simulink model "HANcoder_E407_GTSync_v3_clean"  (R2018b)
settings: Solver=FixedStepDiscrete  StartTime=0.0  StopTime=1  FixedStep=0.01  RelTol=1e-3
PreLoadFcn:
  | librarySetup
  | eval([bdroot,'_startup']) %Calling [modelName]_startup.m
values from neighbouring files (symbols this model uses):
  basic_cycle_duration = 60000    [HANcoder_E407_GTSync_v3_clean_startup.m]    (also in HANcoder_E407_GTSync_v3_startup.m = 50000)
  comm_delay_estimation = 3    [HANcoder_E407_GTSync_v3_clean_startup.m]
  frequency_IRQ = 100    [HANcoder_E407_GTSync_startup.m]    (also in HANcoder_E407_GTSync_v3_clean_startup.m = 99; HANcoder_E407_GTSync_v3_startup.m = 99)
  HANtuneOverride = Simulink.Parameter    [HANcoder_E407_GTSync_startup.m]    (also in HANcoder_E407_GTSync_v3_clean_startup.m; HANcoder_E407_GTSync_v3_startup.m)
  LED_ticks_toggle = 10000    [HANcoder_E407_GTSync_startup.m]    (also in HANcoder_E407_GTSync_v3_clean_startup.m; HANcoder_E407_GTSync_v3_startup.m)
  Master_Role = 1    [HANcoder_E407_GTSync_v3_clean_startup.m]    (also in HANcoder_E407_GTSync_v3_startup.m)
  matrix_rows = 2    [HANcoder_E407_GTSync_v3_clean_startup.m]    (also in HANcoder_E407_GTSync_v3_startup.m)
  Slave_Role = 2    [HANcoder_E407_GTSync_v3_clean_startup.m]    (also in HANcoder_E407_GTSync_v3_startup.m)
  Sync_ID = 1    [HANcoder_E407_GTSync_v3_clean_startup.m]    (also in HANcoder_E407_GTSync_v3_startup.m)
  time_difference_threshold = 500    [HANcoder_E407_GTSync_v3_clean_startup.m]    (also in HANcoder_E407_GTSync_v3_startup.m = 100)
  TM0 = 100    [HANcoder_E407_GTSync_v3_clean_startup.m]    (also in HANcoder_E407_GTSync_v3_startup.m = 0)
  TM1 = 20000    [HANcoder_E407_GTSync_v3_clean_startup.m]    (also in HANcoder_E407_GTSync_v3_startup.m = 25000)
  TM2 = 30000    [HANcoder_E407_GTSync_v3_clean_startup.m]    (also in HANcoder_E407_GTSync_v3_startup.m = 37500)
  TM3 = 40000    [HANcoder_E407_GTSync_v3_clean_startup.m]    (also in HANcoder_E407_GTSync_v3_startup.m)
  TM4 = 50000    [HANcoder_E407_GTSync_v3_clean_startup.m]
  Vote1_ID = 12    [HANcoder_E407_GTSync_v3_clean_startup.m]    (also in HANcoder_E407_GTSync_v3_startup.m)
  Vote2_ID = 22    [HANcoder_E407_GTSync_v3_clean_startup.m]    (also in HANcoder_E407_GTSync_v3_startup.m)
  Vote3_ID = 32    [HANcoder_E407_GTSync_v3_clean_startup.m]    (also in HANcoder_E407_GTSync_v3_startup.m)
  wrap_up_threshold = basic_cycle_duration - time_difference_threshold*10    (= 55000)    [HANcoder_E407_GTSync_v3_clean_startup.m]
libraries: HANcoder_STM32_Target x20, simulink x3, simulink_extras x1
(part 3 of 4)

== system HANcoder_E407_GTSync_v3_clean/HANcoder STM32 Target - E407-STM32 algorithm/Global Ticks Increment/CAN Management/CAN Recieve/CAN Receive System/Subsystem3 ==
  Enable : EnablePort
  Bus Creator : BusCreator  Inputs=9
  CAN receive : Subsystem  Tag=HANcoder_TARGET_STM32_E407  AncestorBlock=HANcoder_STM32_Target/STM32-E407/CAN/CAN/CAN receive  mask(CAN receive){canBus=CAN 2, outputNumber=8, dataType=uint8, byteOrder=off, tsamp=-1}
      mask prompts: canBus "CAN channel"; outputNumber "Output ports"; dataType "Output datatype"; byteOrder "Byte order: Checked = MSB first, unchecked = LSB first."; tsamp "Sample time"
      mask help:
      | Function
      | ==========
      | Receive the newest message from the specified CAN channel.
      |
      | Parameters
      | ==========
      | CAN channel:             The CAN channel to send the message on.
      | Output ports:             The amount of output ports
      | Output datatype:       The datatype of the output ports
      | Byte order:                 Select MSB or LSB first
      | Sample time:              -1 or divisible by base sample time [seconds]
      |
      | Input
      | ==========
      | Port 1:                       CAN ID(uint32) in hexadecimal ie: hex2dec('0a')
      |
      | Output
      | ==========
      | Port 1:                       Checks for new message(int8)
      | Port 2..9                     Message data
      mask init:
      | sfcn_can_receive_mcb(canBus, outputNumber, dataType, byteOrder)
      settings: MoveFcn=drawLogos
      mask Help: web('sfcn_can_receive.html');
      mask TypeOptions canBus: CAN 1 | CAN 2
      mask TypeOptions dataType: int8 | uint8 | int16 | uint16 | int32 | uint32 | boolean
      mask Display:
      | fprintf('Receive on\nCAN %x', canBus);
      | port_label('output', 1, 'new');
      | port_label('input', 1, 'ID');patch([85 91 91],[8 14 2],[1 0 0]);patch([93 93 99],[14 2 8],[0 0 0.35]);
  Constant4 : Constant  Value=Vote3_ID  OutDataTypeStr=uint32
  Output : Outport
  wires:
  Constant4/1 -> CAN receive/1(In1)
  Bus Creator/1 -> Output/1
  CAN receive/1(Out1) -> Bus Creator/1
  CAN receive/9(Out9) -> Bus Creator/9
  CAN receive/8(Out8) -> Bus Creator/8
  CAN receive/7(Out7) -> Bus Creator/7
  CAN receive/6(Out6) -> Bus Creator/6
  CAN receive/5(Out5) -> Bus Creator/5
  CAN receive/4(Out4) -> Bus Creator/4
  CAN receive/3(Out3) -> Bus Creator/3
  CAN receive/2(Out2) -> Bus Creator/2

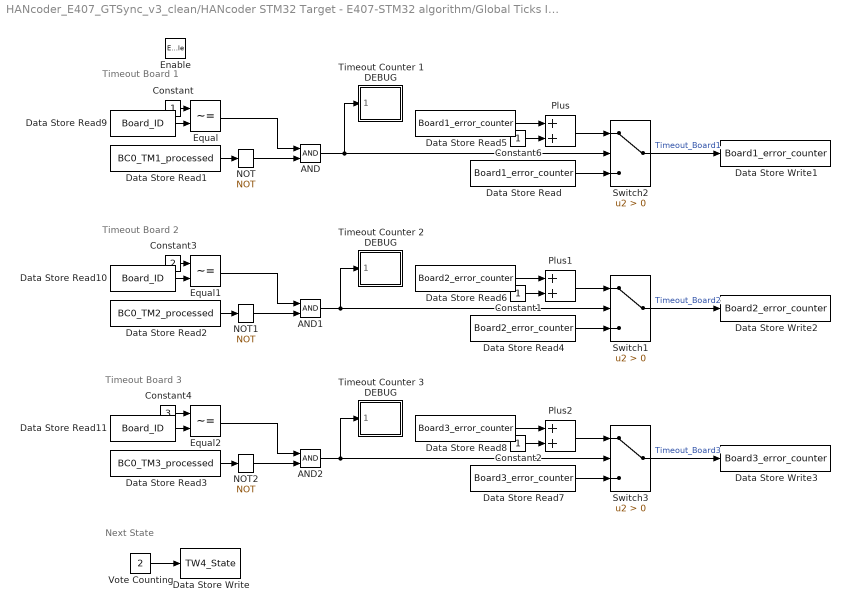
== system HANcoder_E407_GTSync_v3_clean/HANcoder STM32 Target - E407-STM32 algorithm/Global Ticks Increment/CAN Management/Matrix Cycle Manager/BC0 TW4/Subsystem ==
  note: Timeout Board 3
  note: Timeout Board 2
  note: Timeout Board 1
  note: Next State
  Enable : EnablePort
  AND : Logic  IconShape=distinctive  AllPortsSameDT=off  OutDataTypeStr=boolean
  AND1 : Logic  IconShape=distinctive  AllPortsSameDT=off  OutDataTypeStr=boolean
  AND2 : Logic  IconShape=distinctive  AllPortsSameDT=off  OutDataTypeStr=boolean
  Constant{,1..2,6} (4 alike) : Constant
  Constant3 : Constant  Value=2
  Constant4 : Constant  Value=3
  Data Store Read : DataStoreRead  DataStoreName=Board1_error_counter
  Data Store Read1 : DataStoreRead  DataStoreName=BC0_TM1_processed
  Data Store Read10 : DataStoreRead  DataStoreName=Board_ID
  Data Store Read11 : DataStoreRead  DataStoreName=Board_ID
  Data Store Read2 : DataStoreRead  DataStoreName=BC0_TM2_processed
  Data Store Read3 : DataStoreRead  DataStoreName=BC0_TM3_processed
  Data Store Read4 : DataStoreRead  DataStoreName=Board2_error_counter
  Data Store Read5 : DataStoreRead  DataStoreName=Board1_error_counter
  Data Store Read6 : DataStoreRead  DataStoreName=Board2_error_counter
  Data Store Read7 : DataStoreRead  DataStoreName=Board3_error_counter
  Data Store Read8 : DataStoreRead  DataStoreName=Board3_error_counter
  Data Store Read9 : DataStoreRead  DataStoreName=Board_ID
  Data Store Write : DataStoreWrite  DataStoreName=TW4_State
  Data Store Write1 : DataStoreWrite  DataStoreName=Board1_error_counter
  Data Store Write2 : DataStoreWrite  DataStoreName=Board2_error_counter
  Data Store Write3 : DataStoreWrite  DataStoreName=Board3_error_counter
  Equal : RelationalOperator  Operator=~=  OutDataTypeStr=boolean  RndMeth=Simplest
  Equal1 : RelationalOperator  Operator=~=  OutDataTypeStr=boolean  RndMeth=Simplest
  Equal2 : RelationalOperator  Operator=~=  OutDataTypeStr=boolean  RndMeth=Simplest
  NOT : Logic  Operator=NOT  IconShape=distinctive  AllPortsSameDT=off  OutDataTypeStr=boolean
  NOT1 : Logic  Operator=NOT  IconShape=distinctive  AllPortsSameDT=off  OutDataTypeStr=boolean
  NOT2 : Logic  Operator=NOT  IconShape=distinctive  AllPortsSameDT=off  OutDataTypeStr=boolean
  Plus : Sum
  Plus1 : Sum
  Plus2 : Sum
  Switch1 : Switch  Criteria=u2 > Threshold
  Switch2 : Switch  Criteria=u2 > Threshold
  Switch3 : Switch  Criteria=u2 > Threshold
  Timeout Counter 1 DEBUG : Subsystem
  Timeout Counter 2 DEBUG : Subsystem
  Timeout Counter 3 DEBUG : Subsystem
  Vote Counting : Constant  Value=2
  wires:
  Vote Counting/1 -> Data Store Write/1
  Constant6/1 -> Plus/2
  Plus/1 -> Switch2/1
  Data Store Read5/1 -> Plus/1
  Switch2/1 -> Data Store Write1/1  "Timeout_Board1"
  Data Store Read/1 -> Switch2/3
  Data Store Read1/1 -> NOT/1
  Data Store Read2/1 -> NOT1/1
  Data Store Read4/1 -> Switch1/3
  Switch1/1 -> Data Store Write2/1  "Timeout_Board2"
  Data Store Read6/1 -> Plus1/1
  Plus1/1 -> Switch1/1
  Constant1/1 -> Plus1/2
  Constant2/1 -> Plus2/2
  Plus2/1 -> Switch3/1
  Switch3/1 -> Data Store Write3/1  "Timeout_Board3"
  Data Store Read7/1 -> Switch3/3
  Data Store Read3/1 -> NOT2/1
  Data Store Read8/1 -> Plus2/1
  NOT/1 -> AND/2
  Data Store Read9/1 -> Equal/2
  Constant/1 -> Equal/1
  Equal/1 -> AND/1
  AND/1 -> Timeout Counter 1 DEBUG/1(Timeout), Switch2/2
  Equal1/1 -> AND1/1
  Equal2/1 -> AND2/1
  NOT2/1 -> AND2/2
  AND2/1 -> Timeout Counter 3 DEBUG/1(Timeout), Switch3/2
  Data Store Read11/1 -> Equal2/2
  Constant4/1 -> Equal2/1
  Data Store Read10/1 -> Equal1/2
  Constant3/1 -> Equal1/1
  AND1/1 -> Timeout Counter 2 DEBUG/1(Timeout), Switch1/2
  NOT1/1 -> AND1/2

== system HANcoder_E407_GTSync_v3_clean/HANcoder STM32 Target - E407-STM32 algorithm/Global Ticks Increment/CAN Management/Matrix Cycle Manager/BC0 TW4/Subsystem2 ==
  note: Next State
  note: Post voting process
  Enable : EnablePort  PropagateVarSize=During execution
  Constant10 : Constant  Value=Slave_Role
  Constant9 : Constant  Value=Master_Role
  Data Store Read : DataStoreRead  DataStoreName=Master_ID
  Data Store Read27 : DataStoreRead  DataStoreName=Board_ID
  Data Store Write : DataStoreWrite  DataStoreName=TW4_State
  Data Store Write1 : DataStoreWrite  DataStoreName=New_Master
  Data Store Write13 : DataStoreWrite  DataStoreName=Master_ID
  Data Store Write15 : DataStoreWrite  DataStoreName=Role_ID
  Equal : RelationalOperator  Operator=~=  OutDataTypeStr=boolean  RndMeth=Simplest
  Equal6 : RelationalOperator  Operator===  OutDataTypeStr=boolean  RndMeth=Simplest
  RESET Board - Return to initialization : Subsystem  TreatAsAtomicUnit=on
  Reset Variables : Constant  Value=3
  Switch16 : Switch  Criteria=u2 > Threshold
  Votes recount to choose Master : Subsystem
  wires:
  Reset Variables/1 -> Data Store Write/1
  Equal6/1 -> Switch16/2
  Data Store Read27/1 -> Equal6/2
  Switch16/1 -> Data Store Write15/1  "Role_ID_s"
  Constant9/1 -> Switch16/1
  Constant10/1 -> Switch16/3
  Data Store Read/1 -> Equal/1
  Equal/1 -> Data Store Write1/1
  Votes recount to choose Master/1(Master_ID_s) -> Equal6/1, Equal/2, Data Store Write13/1
  Votes recount to choose Master/2(Reset Board) -> RESET Board - Return to initialization/Enable

== system HANcoder_E407_GTSync_v3_clean/HANcoder STM32 Target - E407-STM32 algorithm/Global Ticks Increment/CAN Management/Matrix Cycle Manager/BC0 TW4/Subsystem3 ==
  note: Next State
  note: Reset variables
  Enable : EnablePort
  Cast : DataTypeConversion  OutDataTypeStr=boolean
  Constant : Constant  Value=0
  Data Store Write : DataStoreWrite  DataStoreName=TW4_State
  Data Store Write1 : DataStoreWrite  DataStoreName=sync_processed
  Data Store Write16 : DataStoreWrite  DataStoreName=votes  DataStoreElements=votes.First_Board#votes.Second_Board#votes.Third_Board
  Data Store Write2 : DataStoreWrite  DataStoreName=BC0_TM1_processed
  Data Store Write3 : DataStoreWrite  DataStoreName=BC0_TM2_processed
  Data Store Write4 : DataStoreWrite  DataStoreName=BC0_TM3_processed
  Finished : Constant  Value=4
  Reset TW1 State : DataStoreWrite  DataStoreName=TW1_State
  Vote time : Constant
  wires:
  Finished/1 -> Data Store Write/1
  Constant/1 -> Data Store Write16/1, Cast/1, Data Store Write16/3, Data Store Write16/2
  Vote time/1 -> Reset TW1 State/1
  Cast/1 -> Data Store Write4/1, Data Store Write3/1, Data Store Write2/1, Data Store Write1/1

== system HANcoder_E407_GTSync_v3_clean/HANcoder STM32 Target - E407-STM32 algorithm/Global Ticks Increment/CAN Management/Matrix Cycle Manager/BC1 TW4/Subsystem3 ==
  note: Reset variables
  note: Next State
  Enable : EnablePort
  Cast : DataTypeConversion  OutDataTypeStr=boolean
  Constant : Constant  Value=0
  Data Store Write : DataStoreWrite  DataStoreName=TW4_State
  Data Store Write1 : DataStoreWrite  DataStoreName=sync_processed
  Finished : Constant
  wires:
  Cast/1 -> Data Store Write1/1
  Constant/1 -> Cast/1
  Finished/1 -> Data Store Write/1

== system HANcoder_E407_GTSync_v3_clean/HANcoder STM32 Target - E407-STM32 algorithm/Global Ticks Increment/CAN Management/Matrix Cycle Manager/Local Time Update/Process Time Difference ==
  Rx_Time : Inport
  Local_Time : Inport  Port=2
  Check_Wrap_up : Subsystem
  Check_Wrap_up1 : Subsystem
  Minus : Sum  Inputs=+-
  Time_Difference : Outport
  wires:
  Minus/1 -> Time_Difference/1
  Rx_Time/1 -> Check_Wrap_up/1(In1)
  Local_Time/1 -> Check_Wrap_up1/1(In1)
  Check_Wrap_up/1(Out1) -> Minus/1
  Check_Wrap_up1/1(Out1) -> Minus/2

== system HANcoder_E407_GTSync_v3_clean/HANcoder STM32 Target - E407-STM32 algorithm/Global Ticks Increment/CAN Management/Matrix Cycle Manager/Local Time Update/Time_Difference_DEBUG ==
  RXID : Inport
  Time_Difference : Inport  Port=2
  Constant : Constant  Value=Vote1_ID
  Constant1 : Constant  Value=Vote2_ID
  Constant2 : Constant  Value=Vote3_ID
  Constant3 : Constant  Value=Sync_ID
  Data Store Read : DataStoreRead  DataStoreName=time_difference_sync
  Data Store Read1 : DataStoreRead  DataStoreName=time_difference_vote1
  Data Store Read2 : DataStoreRead  DataStoreName=time_difference_vote2
  Data Store Read3 : DataStoreRead  DataStoreName=time_difference_vote3
  Data Store Write : DataStoreWrite  DataStoreName=time_difference_sync
  Data Store Write1 : DataStoreWrite  DataStoreName=time_difference_vote1
  Data Store Write2 : DataStoreWrite  DataStoreName=time_difference_vote2
  Data Store Write3 : DataStoreWrite  DataStoreName=time_difference_vote3
  Equal{,1..3} (4 alike) : RelationalOperator  Operator===  OutDataTypeStr=boolean  RndMeth=Simplest
  Switch{,1..3} (4 alike) : Switch  Criteria=u2 > Threshold
  wires:
  Time_Difference/1 -> Switch/1, Switch1/1, Switch2/1, Switch3/1
  Constant3/1 -> Equal/1
  Constant/1 -> Equal1/1
  Constant1/1 -> Equal2/1
  Constant2/1 -> Equal3/1
  RXID/1 -> Equal3/2, Equal2/2, Equal1/2, Equal/2
  Equal/1 -> Switch/2
  Equal1/1 -> Switch1/2
  Equal2/1 -> Switch2/2
  Switch/1 -> Data Store Write/1  "time_difference_sync_s"
  Switch1/1 -> Data Store Write1/1  "time_difference_vote1_s"
  Switch2/1 -> Data Store Write2/1  "time_difference_vote2_s"
  Equal3/1 -> Switch3/2
  Switch3/1 -> Data Store Write3/1  "time_difference_vote3_s"
  Data Store Read/1 -> Switch/3
  Data Store Read1/1 -> Switch1/3
  Data Store Read2/1 -> Switch2/3
  Data Store Read3/1 -> Switch3/3

== system HANcoder_E407_GTSync_v3_clean/HANcoder STM32 Target - E407-STM32 algorithm/Global Ticks Increment/CAN Management/Matrix Cycle Manager/Vote Count 1/Sum up new vote ==
  note: Registering votes
  Msg Header : Inport
  Enable : EnablePort
  Add : Sum
  Add1 : Sum
  Add2 : Sum
  Constant10 : Constant
  Constant11 : Constant  Value=2
  Constant12 : Constant  Value=3
  Data Store Read15 : DataStoreRead  DataStoreName=votes  DataStoreElements=votes.First_Board
  Data Store Read16 : DataStoreRead  DataStoreName=votes  DataStoreElements=votes.Second_Board
  Data Store Read17 : DataStoreRead  DataStoreName=votes  DataStoreElements=votes.Third_Board
  Data Store Write12 : DataStoreWrite  DataStoreName=votes  DataStoreElements=votes.First_Board#votes.Second_Board#votes.Third_Board
  Equal13 : RelationalOperator  Operator===  OutDataTypeStr=boolean  RndMeth=Simplest
  Equal15 : RelationalOperator  Operator===  OutDataTypeStr=boolean  RndMeth=Simplest
  Equal17 : RelationalOperator  Operator===  OutDataTypeStr=boolean  RndMeth=Simplest
  wires:
  Equal17/1 -> Add2/2
  Constant12/1 -> Equal17/1
  Add2/1 -> Data Store Write12/3
  Msg Header/1 -> Equal17/2, Equal15/2, Equal13/2
  Constant11/1 -> Equal15/1
  Data Store Read16/1 -> Add1/1
  Data Store Read15/1 -> Add/1
  Equal15/1 -> Add1/2
  Data Store Read17/1 -> Add2/1
  Constant10/1 -> Equal13/1
  Add1/1 -> Data Store Write12/2
  Add/1 -> Data Store Write12/1
  Equal13/1 -> Add/2

== system HANcoder_E407_GTSync_v3_clean/HANcoder STM32 Target - E407-STM32 algorithm/Global Ticks Increment/CAN Management/Matrix Cycle Manager/Vote Count 1/Time_Difference_DEBUG ==
  RXID : Inport
  Time_Difference : Inport  Port=2
  Constant : Constant  Value=Vote1_ID
  Constant1 : Constant  Value=Vote2_ID
  Constant2 : Constant  Value=Vote3_ID
  Constant3 : Constant  Value=Sync_ID
  Data Store Read : DataStoreRead  DataStoreName=time_difference_sync
  Data Store Read1 : DataStoreRead  DataStoreName=time_difference_vote1
  Data Store Read2 : DataStoreRead  DataStoreName=time_difference_vote2
  Data Store Read3 : DataStoreRead  DataStoreName=time_difference_vote3
  Data Store Write : DataStoreWrite  DataStoreName=time_difference_sync
  Data Store Write1 : DataStoreWrite  DataStoreName=time_difference_vote1
  Data Store Write2 : DataStoreWrite  DataStoreName=time_difference_vote2
  Data Store Write3 : DataStoreWrite  DataStoreName=time_difference_vote3
  Equal{,1..3} (4 alike) : RelationalOperator  Operator===  OutDataTypeStr=boolean  RndMeth=Simplest
  Switch{,1..3} (4 alike) : Switch  Criteria=u2 > Threshold
  wires:
  Time_Difference/1 -> Switch/1, Switch1/1, Switch2/1, Switch3/1
  Constant3/1 -> Equal/1
  Constant/1 -> Equal1/1
  Constant1/1 -> Equal2/1
  Constant2/1 -> Equal3/1
  RXID/1 -> Equal3/2, Equal2/2, Equal1/2, Equal/2
  Equal/1 -> Switch/2
  Equal1/1 -> Switch1/2
  Equal2/1 -> Switch2/2
  Switch/1 -> Data Store Write/1  "time_difference_sync_s1"
  Switch1/1 -> Data Store Write1/1  "time_difference_vote1_s1"
  Switch2/1 -> Data Store Write2/1  "time_difference_vote2_s1"
  Equal3/1 -> Switch3/2
  Switch3/1 -> Data Store Write3/1  "time_difference_vote3_s1"
  Data Store Read/1 -> Switch/3
  Data Store Read1/1 -> Switch1/3
  Data Store Read2/1 -> Switch2/3
  Data Store Read3/1 -> Switch3/3

== system HANcoder_E407_GTSync_v3_clean/HANcoder STM32 Target - E407-STM32 algorithm/Global Ticks Increment/CAN Management/Matrix Cycle Manager/Vote Count 2/Sum up new vote ==
  note: Registering votes
  Msg Header : Inport
  Enable : EnablePort
  Add : Sum
  Add1 : Sum
  Add2 : Sum
  Constant10 : Constant
  Constant11 : Constant  Value=2
  Constant12 : Constant  Value=3
  Data Store Read15 : DataStoreRead  DataStoreName=votes  DataStoreElements=votes.First_Board
  Data Store Read16 : DataStoreRead  DataStoreName=votes  DataStoreElements=votes.Second_Board
  Data Store Read17 : DataStoreRead  DataStoreName=votes  DataStoreElements=votes.Third_Board
  Data Store Write12 : DataStoreWrite  DataStoreName=votes  DataStoreElements=votes.First_Board#votes.Second_Board#votes.Third_Board
  Equal13 : RelationalOperator  Operator===  OutDataTypeStr=boolean  RndMeth=Simplest
  Equal15 : RelationalOperator  Operator===  OutDataTypeStr=boolean  RndMeth=Simplest
  Equal17 : RelationalOperator  Operator===  OutDataTypeStr=boolean  RndMeth=Simplest
  wires:
  Equal17/1 -> Add2/2
  Constant12/1 -> Equal17/1
  Add2/1 -> Data Store Write12/3
  Msg Header/1 -> Equal17/2, Equal15/2, Equal13/2
  Constant11/1 -> Equal15/1
  Data Store Read16/1 -> Add1/1
  Data Store Read15/1 -> Add/1
  Equal15/1 -> Add1/2
  Data Store Read17/1 -> Add2/1
  Constant10/1 -> Equal13/1
  Add1/1 -> Data Store Write12/2
  Add/1 -> Data Store Write12/1
  Equal13/1 -> Add/2

== system HANcoder_E407_GTSync_v3_clean/HANcoder STM32 Target - E407-STM32 algorithm/Global Ticks Increment/CAN Management/Matrix Cycle Manager/Vote Count 2/Time_Difference_DEBUG ==
  RXID : Inport
  Time_Difference : Inport  Port=2
  Constant : Constant  Value=Vote1_ID
  Constant1 : Constant  Value=Vote2_ID
  Constant2 : Constant  Value=Vote3_ID
  Constant3 : Constant  Value=Sync_ID
  Data Store Read : DataStoreRead  DataStoreName=time_difference_sync
  Data Store Read1 : DataStoreRead  DataStoreName=time_difference_vote1
  Data Store Read2 : DataStoreRead  DataStoreName=time_difference_vote2
  Data Store Read3 : DataStoreRead  DataStoreName=time_difference_vote3
  Data Store Write : DataStoreWrite  DataStoreName=time_difference_sync
  Data Store Write1 : DataStoreWrite  DataStoreName=time_difference_vote1
  Data Store Write2 : DataStoreWrite  DataStoreName=time_difference_vote2
  Data Store Write3 : DataStoreWrite  DataStoreName=time_difference_vote3
  Equal{,1..3} (4 alike) : RelationalOperator  Operator===  OutDataTypeStr=boolean  RndMeth=Simplest
  Switch{,1..3} (4 alike) : Switch  Criteria=u2 > Threshold
  wires:
  Data Store Read3/1 -> Switch3/3
  Data Store Read2/1 -> Switch2/3
  Data Store Read1/1 -> Switch1/3
  Data Store Read/1 -> Switch/3
  Switch3/1 -> Data Store Write3/1  "time_difference_vote3_s2"
  Equal3/1 -> Switch3/2
  Switch2/1 -> Data Store Write2/1  "time_difference_vote2_s2"
  Switch1/1 -> Data Store Write1/1  "time_difference_vote1_s2"
  Switch/1 -> Data Store Write/1  "time_difference_sync_s2"
  Equal2/1 -> Switch2/2
  Equal1/1 -> Switch1/2
  Equal/1 -> Switch/2
  RXID/1 -> Equal/2, Equal1/2, Equal2/2, Equal3/2
  Constant2/1 -> Equal3/1
  Constant1/1 -> Equal2/1
  Constant/1 -> Equal1/1
  Constant3/1 -> Equal/1
  Time_Difference/1 -> Switch3/1, Switch2/1, Switch1/1, Switch/1

== system HANcoder_E407_GTSync_v3_clean/HANcoder STM32 Target - E407-STM32 algorithm/Global Ticks Increment/CAN Management/Matrix Cycle Manager/Vote Count 3/Sum up new vote ==
  note: Registering votes
  Msg Header : Inport
  Enable : EnablePort
  Add : Sum
  Add1 : Sum
  Add2 : Sum
  Constant10 : Constant
  Constant11 : Constant  Value=2
  Constant12 : Constant  Value=3
  Data Store Read15 : DataStoreRead  DataStoreName=votes  DataStoreElements=votes.First_Board
  Data Store Read16 : DataStoreRead  DataStoreName=votes  DataStoreElements=votes.Second_Board
  Data Store Read17 : DataStoreRead  DataStoreName=votes  DataStoreElements=votes.Third_Board
  Data Store Write12 : DataStoreWrite  DataStoreName=votes  DataStoreElements=votes.First_Board#votes.Second_Board#votes.Third_Board
  Equal13 : RelationalOperator  Operator===  OutDataTypeStr=boolean  RndMeth=Simplest
  Equal15 : RelationalOperator  Operator===  OutDataTypeStr=boolean  RndMeth=Simplest
  Equal17 : RelationalOperator  Operator===  OutDataTypeStr=boolean  RndMeth=Simplest
  wires:
  Equal17/1 -> Add2/2
  Constant12/1 -> Equal17/1
  Add2/1 -> Data Store Write12/3
  Msg Header/1 -> Equal17/2, Equal15/2, Equal13/2
  Constant11/1 -> Equal15/1
  Data Store Read16/1 -> Add1/1
  Data Store Read15/1 -> Add/1
  Equal15/1 -> Add1/2
  Data Store Read17/1 -> Add2/1
  Constant10/1 -> Equal13/1
  Add1/1 -> Data Store Write12/2
  Add/1 -> Data Store Write12/1
  Equal13/1 -> Add/2

== system HANcoder_E407_GTSync_v3_clean/HANcoder STM32 Target - E407-STM32 algorithm/Global Ticks Increment/CAN Management/Matrix Cycle Manager/Vote Count 3/Time_Difference_DEBUG ==
  RXID : Inport
  Time_Difference : Inport  Port=2
  Constant : Constant  Value=Vote1_ID
  Constant1 : Constant  Value=Vote2_ID
  Constant2 : Constant  Value=Vote3_ID
  Constant3 : Constant  Value=Sync_ID
  Data Store Read : DataStoreRead  DataStoreName=time_difference_sync
  Data Store Read1 : DataStoreRead  DataStoreName=time_difference_vote1
  Data Store Read2 : DataStoreRead  DataStoreName=time_difference_vote2
  Data Store Read3 : DataStoreRead  DataStoreName=time_difference_vote3
  Data Store Write : DataStoreWrite  DataStoreName=time_difference_sync
  Data Store Write1 : DataStoreWrite  DataStoreName=time_difference_vote1
  Data Store Write2 : DataStoreWrite  DataStoreName=time_difference_vote2
  Data Store Write3 : DataStoreWrite  DataStoreName=time_difference_vote3
  Equal{,1..3} (4 alike) : RelationalOperator  Operator===  OutDataTypeStr=boolean  RndMeth=Simplest
  Switch{,1..3} (4 alike) : Switch  Criteria=u2 > Threshold
  wires:
  Time_Difference/1 -> Switch/1, Switch1/1, Switch2/1, Switch3/1
  Constant3/1 -> Equal/1
  Constant/1 -> Equal1/1
  Constant1/1 -> Equal2/1
  Constant2/1 -> Equal3/1
  RXID/1 -> Equal3/2, Equal2/2, Equal1/2, Equal/2
  Equal/1 -> Switch/2
  Equal1/1 -> Switch1/2
  Equal2/1 -> Switch2/2
  Switch/1 -> Data Store Write/1  "time_difference_sync_s3"
  Switch1/1 -> Data Store Write1/1  "time_difference_vote1_s3"
  Switch2/1 -> Data Store Write2/1  "time_difference_vote2_s3"
  Equal3/1 -> Switch3/2
  Switch3/1 -> Data Store Write3/1  "time_difference_vote3_s3"
  Data Store Read/1 -> Switch/3
  Data Store Read1/1 -> Switch1/3
  Data Store Read2/1 -> Switch2/3
  Data Store Read3/1 -> Switch3/3

== system HANcoder_E407_GTSync_v3_clean/HANcoder STM32 Target - E407-STM32 algorithm/Global Ticks Increment/CAN Management/Matrix Cycle Manager/Vote Decision/Ensure no self votes or failed master reelected ==
  Node ID : Inport
  Sync Timeout : Inport  Port=2
  Error counter : Inport  Port=3
  AND : Logic  IconShape=distinctive  AllPortsSameDT=off  OutDataTypeStr=boolean
  Data Store Read : DataStoreRead  DataStoreName=Board_ID
  Data Store Read2 : DataStoreRead  DataStoreName=Master_ID
  Equal1 : RelationalOperator  Operator===  OutDataTypeStr=boolean  RndMeth=Simplest
  Equal2 : RelationalOperator  Operator===  OutDataTypeStr=boolean  RndMeth=Simplest
  MAX error count : Constant  Value=4294967295  OutDataTypeStr=uint32
  NOT : Logic  Operator=NOT  IconShape=distinctive  AllPortsSameDT=off  OutDataTypeStr=boolean
  OR : Logic  Operator=OR  IconShape=distinctive  AllPortsSameDT=off  OutDataTypeStr=boolean
  Switch : Switch  Criteria=u2 > Threshold
  Out1 : Outport
  wires:
  Equal1/1 -> OR/1
  Data Store Read/1 -> Equal1/2
  MAX error count/1 -> Switch/1
  Switch/1 -> Out1/1
  Error counter/1 -> Switch/3
  Node ID/1 -> Equal1/1, Equal2/2
  Sync Timeout/1 -> NOT/1
  Data Store Read2/1 -> Equal2/1
  Equal2/1 -> AND/1
  NOT/1 -> AND/2
  AND/1 -> OR/2
  OR/1 -> Switch/2

== system HANcoder_E407_GTSync_v3_clean/HANcoder STM32 Target - E407-STM32 algorithm/Global Ticks Increment/CAN Management/Matrix Cycle Manager/Vote Decision/Ensure no self votes or failed master reelected1 ==
  Node ID : Inport
  Sync Timeout : Inport  Port=2
  Error counter : Inport  Port=3
  AND : Logic  IconShape=distinctive  AllPortsSameDT=off  OutDataTypeStr=boolean
  Data Store Read : DataStoreRead  DataStoreName=Board_ID
  Data Store Read2 : DataStoreRead  DataStoreName=Master_ID
  Equal1 : RelationalOperator  Operator===  OutDataTypeStr=boolean  RndMeth=Simplest
  Equal2 : RelationalOperator  Operator===  OutDataTypeStr=boolean  RndMeth=Simplest
  MAX error count : Constant  Value=4294967295  OutDataTypeStr=uint32
  NOT : Logic  Operator=NOT  IconShape=distinctive  AllPortsSameDT=off  OutDataTypeStr=boolean
  OR : Logic  Operator=OR  IconShape=distinctive  AllPortsSameDT=off  OutDataTypeStr=boolean
  Switch : Switch  Criteria=u2 > Threshold
  Out1 : Outport
  wires:
  OR/1 -> Switch/2
  AND/1 -> OR/2
  NOT/1 -> AND/2
  Equal2/1 -> AND/1
  Data Store Read2/1 -> Equal2/1
  Sync Timeout/1 -> NOT/1
  Node ID/1 -> Equal2/2, Equal1/1
  Error counter/1 -> Switch/3
  Switch/1 -> Out1/1
  MAX error count/1 -> Switch/1
  Data Store Read/1 -> Equal1/2
  Equal1/1 -> OR/1

== system HANcoder_E407_GTSync_v3_clean/HANcoder STM32 Target - E407-STM32 algorithm/Global Ticks Increment/CAN Management/Matrix Cycle Manager/Vote Decision/Ensure no self votes or failed master reelected2 ==
  Node ID : Inport
  Sync Timeout : Inport  Port=2
  Error counter : Inport  Port=3
  AND : Logic  IconShape=distinctive  AllPortsSameDT=off  OutDataTypeStr=boolean
  Data Store Read : DataStoreRead  DataStoreName=Board_ID
  Data Store Read2 : DataStoreRead  DataStoreName=Master_ID
  Equal1 : RelationalOperator  Operator===  OutDataTypeStr=boolean  RndMeth=Simplest
  Equal2 : RelationalOperator  Operator===  OutDataTypeStr=boolean  RndMeth=Simplest
  MAX error count : Constant  Value=4294967295  OutDataTypeStr=uint32
  NOT : Logic  Operator=NOT  IconShape=distinctive  AllPortsSameDT=off  OutDataTypeStr=boolean
  OR : Logic  Operator=OR  IconShape=distinctive  AllPortsSameDT=off  OutDataTypeStr=boolean
  Switch : Switch  Criteria=u2 > Threshold
  Out1 : Outport
  wires:
  Equal1/1 -> OR/1
  Data Store Read/1 -> Equal1/2
  MAX error count/1 -> Switch/1
  Switch/1 -> Out1/1
  Error counter/1 -> Switch/3
  Node ID/1 -> Equal1/1, Equal2/2
  Sync Timeout/1 -> NOT/1
  Data Store Read2/1 -> Equal2/1
  Equal2/1 -> AND/1
  NOT/1 -> AND/2
  AND/1 -> OR/2
  OR/1 -> Switch/2

== system HANcoder_E407_GTSync_v3_clean/HANcoder STM32 Target - E407-STM32 algorithm/Global Ticks Increment/CAN Management/CAN Recieve/CAN Receive System/Initialize message reception/Init_CAN_RX ==
  note: Subsystem States:
      | 	1. Collect current msg
      | 	2. Wait for new msg
  Bus Creator : BusCreator  Inputs=8  OutDataTypeStr=Bus: msg_buffer_type
  CAN receive : Subsystem  Tag=HANcoder_TARGET_STM32_E407  AncestorBlock=HANcoder_STM32_Target/STM32-E407/CAN/CAN/CAN receive  mask(CAN receive){canBus=CAN 2, outputNumber=8, dataType=uint8, byteOrder=off, tsamp=-1}
      mask prompts: canBus "CAN channel"; outputNumber "Output ports"; dataType "Output datatype"; byteOrder "Byte order: Checked = MSB first, unchecked = LSB first."; tsamp "Sample time"
      mask help:
      | Function
      | ==========
      | Receive the newest message from the specified CAN channel.
      |
      | Parameters
      | ==========
      | CAN channel:             The CAN channel to send the message on.
      | Output ports:             The amount of output ports
      | Output datatype:       The datatype of the output ports
      | Byte order:                 Select MSB or LSB first
      | Sample time:              -1 or divisible by base sample time [seconds]
      |
      | Input
      | ==========
      | Port 1:                       CAN ID(uint32) in hexadecimal ie: hex2dec('0a')
      |
      | Output
      | ==========
      | Port 1:                       Checks for new message(int8)
      | Port 2..9                     Message data
      mask init:
      | sfcn_can_receive_mcb(canBus, outputNumber, dataType, byteOrder)
      settings: MoveFcn=drawLogos
      mask Help: web('sfcn_can_receive.html');
      mask TypeOptions canBus: CAN 1 | CAN 2
      mask TypeOptions dataType: int8 | uint8 | int16 | uint16 | int32 | uint32 | boolean
      mask Display:
      | fprintf('Receive on\nCAN %x', canBus);
      | port_label('output', 1, 'new');
      | port_label('input', 1, 'ID');patch([85 91 91],[8 14 2],[1 0 0]);patch([93 93 99],[14 2 8],[0 0 0.35]);
  Constant : Constant  Value=Sync_ID  OutDataTypeStr=uint32
  Constant1 : Constant
  Constant2 : Constant  Value=2
  Data Store Read1 : DataStoreRead  DataStoreName=Init_CAN_RX_State
  Data Store Read2 : DataStoreRead  DataStoreName=Init_CAN_RX_State
  Equal : RelationalOperator  Operator===  OutDataTypeStr=boolean  RndMeth=Simplest
  Equal1 : RelationalOperator  Operator===  OutDataTypeStr=boolean  RndMeth=Simplest
  NOT : Logic  Operator=NOT  IconShape=distinctive  AllPortsSameDT=off  OutDataTypeStr=boolean
  OR : Logic  Operator=OR  IconShape=distinctive  AllPortsSameDT=off  OutDataTypeStr=boolean
  Subsystem : Subsystem
  Subsystem1 : Subsystem
  Init CAN : Outport
  wires:
  CAN receive/5(Out5) -> Bus Creator/4
  CAN receive/2(Out2) -> Bus Creator/1
  CAN receive/8(Out8) -> Bus Creator/7
  Constant/1 -> CAN receive/1(In1)
  CAN receive/9(Out9) -> Bus Creator/8
  CAN receive/3(Out3) -> Bus Creator/2
  CAN receive/7(Out7) -> Bus Creator/6
  CAN receive/4(Out4) -> Bus Creator/3
  CAN receive/6(Out6) -> Bus Creator/5
  CAN receive/1(Out1) -> NOT/1
  Bus Creator/1 -> Subsystem/1(Initial Msg), Subsystem1/1(Current Msg)
  Data Store Read1/1 -> Equal/1
  Constant1/1 -> Equal/2
  Equal/1 -> Subsystem/Enable
  Equal1/1 -> Subsystem1/Enable
  Constant2/1 -> Equal1/2
  Data Store Read2/1 -> Equal1/1
  NOT/1 -> OR/1
  Subsystem1/1(New and Different Msg) -> OR/2
  OR/1 -> Init CAN/1

== system HANcoder_E407_GTSync_v3_clean/HANcoder STM32 Target - E407-STM32 algorithm/Global Ticks Increment/CAN Management/CAN Recieve/CAN Receive System/Subsystem/CAN receive ==
  In1 : Inport
  Enabled Subsystem : Subsystem  TreatAsAtomicUnit=on
  S-Function : M-S-Function  FunctionName=sfcn_can_receive  Parameters=tsamp, canBus, outputNumber, dataType, byteOrder
  Out1 : Outport
  Out2 : Outport  Port=2
  Out3 : Outport  Port=3
  Out4 : Outport  Port=4
  Out5 : Outport  Port=5
  Out6 : Outport  Port=6
  Out7 : Outport  Port=7
  Out8 : Outport  Port=8
  Out9 : Outport  Port=9
  wires:
  S-Function/9 -> Enabled Subsystem/8(In8)
  S-Function/4 -> Enabled Subsystem/3(In3)
  S-Function/5 -> Enabled Subsystem/4(In4)
  S-Function/8 -> Enabled Subsystem/7(In7)
  S-Function/7 -> Enabled Subsystem/6(In6)
  S-Function/6 -> Enabled Subsystem/5(In5)
  Enabled Subsystem/8(Out8) -> Out9/1
  Enabled Subsystem/7(Out7) -> Out8/1
  Enabled Subsystem/6(Out6) -> Out7/1
  Enabled Subsystem/5(Out5) -> Out6/1
  Enabled Subsystem/4(Out4) -> Out5/1
  Enabled Subsystem/3(Out3) -> Out4/1
  Enabled Subsystem/2(Out2) -> Out3/1
  Enabled Subsystem/1(Out1) -> Out2/1
  S-Function/3 -> Enabled Subsystem/2(In2)
  S-Function/2 -> Enabled Subsystem/1(In1)
  S-Function/1 -> Out1/1, Enabled Subsystem/Enable
  In1/1 -> S-Function/1

== system HANcoder_E407_GTSync_v3_clean/HANcoder STM32 Target - E407-STM32 algorithm/Global Ticks Increment/CAN Management/CAN Recieve/CAN Receive System/Subsystem1/CAN receive ==
  In1 : Inport
  Enabled Subsystem : Subsystem  TreatAsAtomicUnit=on
  S-Function : M-S-Function  FunctionName=sfcn_can_receive  Parameters=tsamp, canBus, outputNumber, dataType, byteOrder
  Out1 : Outport
  Out2 : Outport  Port=2
  Out3 : Outport  Port=3
  Out4 : Outport  Port=4
  Out5 : Outport  Port=5
  Out6 : Outport  Port=6
  Out7 : Outport  Port=7
  Out8 : Outport  Port=8
  Out9 : Outport  Port=9
  wires:
  In1/1 -> S-Function/1
  S-Function/1 -> Enabled Subsystem/Enable, Out1/1
  S-Function/2 -> Enabled Subsystem/1(In1)
  S-Function/3 -> Enabled Subsystem/2(In2)
  Enabled Subsystem/1(Out1) -> Out2/1
  Enabled Subsystem/2(Out2) -> Out3/1
  Enabled Subsystem/3(Out3) -> Out4/1
  Enabled Subsystem/4(Out4) -> Out5/1
  Enabled Subsystem/5(Out5) -> Out6/1
  Enabled Subsystem/6(Out6) -> Out7/1
  Enabled Subsystem/7(Out7) -> Out8/1
  Enabled Subsystem/8(Out8) -> Out9/1
  S-Function/6 -> Enabled Subsystem/5(In5)
  S-Function/7 -> Enabled Subsystem/6(In6)
  S-Function/8 -> Enabled Subsystem/7(In7)
  S-Function/5 -> Enabled Subsystem/4(In4)
  S-Function/4 -> Enabled Subsystem/3(In3)
  S-Function/9 -> Enabled Subsystem/8(In8)

== system HANcoder_E407_GTSync_v3_clean/HANcoder STM32 Target - E407-STM32 algorithm/Global Ticks Increment/CAN Management/CAN Recieve/CAN Receive System/Subsystem2/CAN receive ==
  In1 : Inport
  Enabled Subsystem : Subsystem  TreatAsAtomicUnit=on
  S-Function : M-S-Function  FunctionName=sfcn_can_receive  Parameters=tsamp, canBus, outputNumber, dataType, byteOrder
  Out1 : Outport
  Out2 : Outport  Port=2
  Out3 : Outport  Port=3
  Out4 : Outport  Port=4
  Out5 : Outport  Port=5
  Out6 : Outport  Port=6
  Out7 : Outport  Port=7
  Out8 : Outport  Port=8
  Out9 : Outport  Port=9
  wires:
  S-Function/9 -> Enabled Subsystem/8(In8)
  S-Function/4 -> Enabled Subsystem/3(In3)
  S-Function/5 -> Enabled Subsystem/4(In4)
  S-Function/8 -> Enabled Subsystem/7(In7)
  S-Function/7 -> Enabled Subsystem/6(In6)
  S-Function/6 -> Enabled Subsystem/5(In5)
  Enabled Subsystem/8(Out8) -> Out9/1
  Enabled Subsystem/7(Out7) -> Out8/1
  Enabled Subsystem/6(Out6) -> Out7/1
  Enabled Subsystem/5(Out5) -> Out6/1
  Enabled Subsystem/4(Out4) -> Out5/1
  Enabled Subsystem/3(Out3) -> Out4/1
  Enabled Subsystem/2(Out2) -> Out3/1
  Enabled Subsystem/1(Out1) -> Out2/1
  S-Function/3 -> Enabled Subsystem/2(In2)
  S-Function/2 -> Enabled Subsystem/1(In1)
  S-Function/1 -> Out1/1, Enabled Subsystem/Enable
  In1/1 -> S-Function/1

== system HANcoder_E407_GTSync_v3_clean/HANcoder STM32 Target - E407-STM32 algorithm/Global Ticks Increment/CAN Management/CAN Recieve/CAN Receive System/Subsystem3/CAN receive ==
  In1 : Inport
  Enabled Subsystem : Subsystem  TreatAsAtomicUnit=on
  S-Function : M-S-Function  FunctionName=sfcn_can_receive  Parameters=tsamp, canBus, outputNumber, dataType, byteOrder
  Out1 : Outport
  Out2 : Outport  Port=2
  Out3 : Outport  Port=3
  Out4 : Outport  Port=4
  Out5 : Outport  Port=5
  Out6 : Outport  Port=6
  Out7 : Outport  Port=7
  Out8 : Outport  Port=8
  Out9 : Outport  Port=9
  wires:
  In1/1 -> S-Function/1
  S-Function/1 -> Enabled Subsystem/Enable, Out1/1
  S-Function/2 -> Enabled Subsystem/1(In1)
  S-Function/3 -> Enabled Subsystem/2(In2)
  Enabled Subsystem/1(Out1) -> Out2/1
  Enabled Subsystem/2(Out2) -> Out3/1
  Enabled Subsystem/3(Out3) -> Out4/1
  Enabled Subsystem/4(Out4) -> Out5/1
  Enabled Subsystem/5(Out5) -> Out6/1
  Enabled Subsystem/6(Out6) -> Out7/1
  Enabled Subsystem/7(Out7) -> Out8/1
  Enabled Subsystem/8(Out8) -> Out9/1
  S-Function/6 -> Enabled Subsystem/5(In5)
  S-Function/7 -> Enabled Subsystem/6(In6)
  S-Function/8 -> Enabled Subsystem/7(In7)
  S-Function/5 -> Enabled Subsystem/4(In4)
  S-Function/4 -> Enabled Subsystem/3(In3)
  S-Function/9 -> Enabled Subsystem/8(In8)

== system HANcoder_E407_GTSync_v3_clean/HANcoder STM32 Target - E407-STM32 algorithm/Global Ticks Increment/CAN Management/Matrix Cycle Manager/BC0 TW4/Subsystem/Timeout Counter 1 DEBUG ==
  Timeout : Inport
  Constant : Constant
  Data Store Memory : DataStoreMemory  DataStoreName=BC0_TM1_timeout_counter  ReadBeforeWriteMsg=warning  WriteAfterWriteMsg=warning  WriteAfterReadMsg=warning  ShowAdditionalParam=off
  Data Store Read : DataStoreRead  DataStoreName=BC0_TM1_timeout_counter
  Data Store Read1 : DataStoreRead  DataStoreName=BC0_TM1_timeout_counter
  Data Store Write : DataStoreWrite  DataStoreName=BC0_TM1_timeout_counter
  Plus : Sum
  Switch : Switch  Criteria=u2 > Threshold
  wires:
  Timeout/1 -> Switch/2
  Switch/1 -> Data Store Write/1  "TM1_timeout_counter_s"
  Data Store Read1/1 -> Plus/1
  Constant/1 -> Plus/2
  Plus/1 -> Switch/1
  Data Store Read/1 -> Switch/3

== system HANcoder_E407_GTSync_v3_clean/HANcoder STM32 Target - E407-STM32 algorithm/Global Ticks Increment/CAN Management/Matrix Cycle Manager/BC0 TW4/Subsystem/Timeout Counter 2 DEBUG ==
  Timeout : Inport
  Constant : Constant
  Data Store Memory : DataStoreMemory  DataStoreName=BC0_TM2_timeout_counter  ReadBeforeWriteMsg=warning  WriteAfterWriteMsg=warning  WriteAfterReadMsg=warning  ShowAdditionalParam=off
  Data Store Read : DataStoreRead  DataStoreName=BC0_TM2_timeout_counter
  Data Store Read1 : DataStoreRead  DataStoreName=BC0_TM2_timeout_counter
  Data Store Write : DataStoreWrite  DataStoreName=BC0_TM2_timeout_counter
  Plus : Sum
  Switch : Switch  Criteria=u2 > Threshold
  wires:
  Data Store Read/1 -> Switch/3
  Plus/1 -> Switch/1
  Constant/1 -> Plus/2
  Data Store Read1/1 -> Plus/1
  Switch/1 -> Data Store Write/1  "TM2_timeout_counter_s"
  Timeout/1 -> Switch/2

== system HANcoder_E407_GTSync_v3_clean/HANcoder STM32 Target - E407-STM32 algorithm/Global Ticks Increment/CAN Management/Matrix Cycle Manager/BC0 TW4/Subsystem/Timeout Counter 3 DEBUG ==
  Timeout : Inport
  Constant : Constant
  Data Store Memory : DataStoreMemory  DataStoreName=BC0_TM3_timeout_counter  ReadBeforeWriteMsg=warning  WriteAfterWriteMsg=warning  WriteAfterReadMsg=warning  ShowAdditionalParam=off
  Data Store Read : DataStoreRead  DataStoreName=BC0_TM3_timeout_counter
  Data Store Read1 : DataStoreRead  DataStoreName=BC0_TM3_timeout_counter
  Data Store Write : DataStoreWrite  DataStoreName=BC0_TM3_timeout_counter
  Plus : Sum
  Switch : Switch  Criteria=u2 > Threshold
  wires:
  Timeout/1 -> Switch/2
  Switch/1 -> Data Store Write/1  "TM3_timeout_counter_s"
  Data Store Read1/1 -> Plus/1
  Constant/1 -> Plus/2
  Plus/1 -> Switch/1
  Data Store Read/1 -> Switch/3

== system HANcoder_E407_GTSync_v3_clean/HANcoder STM32 Target - E407-STM32 algorithm/Global Ticks Increment/CAN Management/Matrix Cycle Manager/BC0 TW4/Subsystem2/RESET Board - Return to initialization ==
  Enable : EnablePort
  Cast : DataTypeConversion  OutDataTypeStr=boolean
  Constant : Constant  Value=0
  Data Store Write : DataStoreWrite  DataStoreName=first_sync_msg_flag
  Data Store Write1 : DataStoreWrite  DataStoreName=Initialization_CAN_flag
  Data Store Write2 : DataStoreWrite  DataStoreName=Initialization_flag
  Data Store Write3 : DataStoreWrite  DataStoreName=Initialization_Counter
  Data Store Write4 : DataStoreWrite  DataStoreName=Role_ID
  Data Store Write5 : DataStoreWrite  DataStoreName=Idle_Time_Finish_Flag
  wires:
  Constant/1 -> Data Store Write4/1, Data Store Write3/1, Cast/1
  Cast/1 -> Data Store Write/1, Data Store Write1/1, Data Store Write5/1, Data Store Write2/1

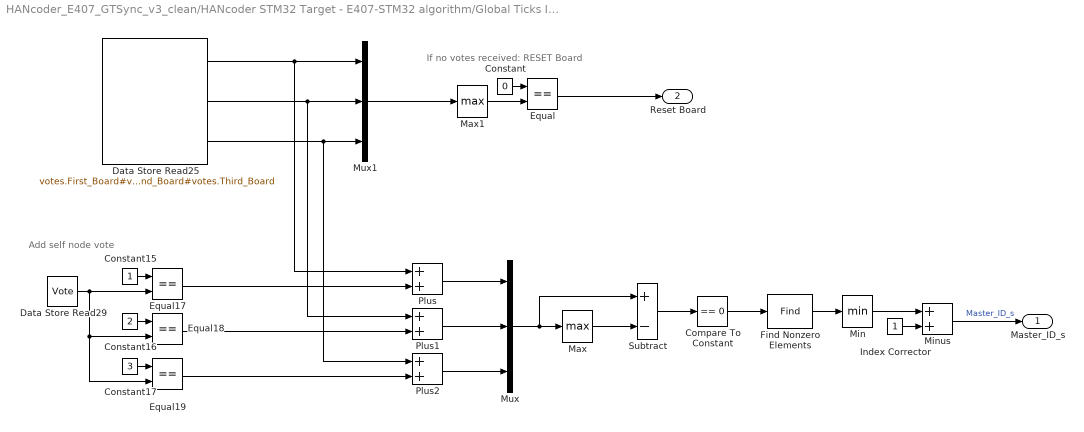
== system HANcoder_E407_GTSync_v3_clean/HANcoder STM32 Target - E407-STM32 algorithm/Global Ticks Increment/CAN Management/Matrix Cycle Manager/BC0 TW4/Subsystem2/Votes recount to choose Master ==
  note: If no votes received: RESET Board
  note: Add self node vote
  Compare To Constant : simulink/Logic and Bit Operations/Compare To Constant  relop===  const=0  OutDataTypeStr=boolean
  Constant : Constant  Value=0
  Constant15 : Constant
  Constant16 : Constant  Value=2
  Constant17 : Constant  Value=3
  Data Store Read25 : DataStoreRead  DataStoreName=votes  DataStoreElements=votes.First_Board#votes.Second_Board#votes.Third_Board
  Data Store Read29 : DataStoreRead  DataStoreName=Vote
  Equal{,17..19} (4 alike) : RelationalOperator  Operator===  OutDataTypeStr=boolean  RndMeth=Simplest
  Find Nonzero Elements : Find  NumberOfInputDimensions=3  IndexMode=Zero-based
  Index Corrector : Constant
  Max : MinMax  Function=max
  Max1 : MinMax  Function=max
  Min : MinMax
  Minus : Sum
  Mux : Mux  Inputs=3
  Mux1 : Mux  Inputs=3
  Plus : Sum
  Plus1 : Sum
  Plus2 : Sum
  Subtract : Sum  Inputs=+-
  Master_ID_s : Outport
  Reset Board : Outport  Port=2
  wires:
  Data Store Read25/1 -> Plus/1, Mux1/1
  Equal18/1 -> Plus1/2
  Plus/1 -> Mux/1
  Constant15/1 -> Equal17/1
  Plus1/1 -> Mux/2
  Min/1 -> Minus/1
  Index Corrector/1 -> Minus/2
  Data Store Read25/2 -> Plus1/1, Mux1/2
  Plus2/1 -> Mux/3
  Equal19/1 -> Plus2/2
  Data Store Read29/1 -> Equal19/2, Equal18/2, Equal17/2
  Find Nonzero Elements/1 -> Min/1
  Equal17/1 -> Plus/2
  Subtract/1 -> Compare To Constant/1
  Constant16/1 -> Equal18/1
  Max/1 -> Subtract/2
  Mux/1 -> Subtract/1, Max/1
  Data Store Read25/3 -> Plus2/1, Mux1/3
  Constant17/1 -> Equal19/1
  Compare To Constant/1 -> Find Nonzero Elements/1
  Minus/1 -> Master_ID_s/1  "Master_ID_s"
  Mux1/1 -> Max1/1
  Max1/1 -> Equal/2
  Constant/1 -> Equal/1
  Equal/1 -> Reset Board/1

== system HANcoder_E407_GTSync_v3_clean/HANcoder STM32 Target - E407-STM32 algorithm/Global Ticks Increment/CAN Management/Matrix Cycle Manager/Local Time Update/Process Time Difference/Check_Wrap_up ==
  In1 : Inport
  GreaterThan : RelationalOperator  Operator=>  OutDataTypeStr=boolean  RndMeth=Simplest
  Minus : Sum  Inputs=+-
  Switch : Switch  Criteria=u2 > Threshold
  Wrap-up_Threshold : Constant  Value=wrap_up_threshold
  Wrap-up_Threshold1 : Constant  Value=basic_cycle_duration
  Out1 : Outport
  wires:
  In1/1 -> Minus/1, Switch/3, GreaterThan/1
  Wrap-up_Threshold/1 -> GreaterThan/2
  GreaterThan/1 -> Switch/2
  Switch/1 -> Out1/1
  Minus/1 -> Switch/1
  Wrap-up_Threshold1/1 -> Minus/2

== system HANcoder_E407_GTSync_v3_clean/HANcoder STM32 Target - E407-STM32 algorithm/Global Ticks Increment/CAN Management/Matrix Cycle Manager/Local Time Update/Process Time Difference/Check_Wrap_up1 ==
  In1 : Inport
  GreaterThan : RelationalOperator  Operator=>  OutDataTypeStr=boolean  RndMeth=Simplest
  Minus : Sum  Inputs=+-
  Switch : Switch  Criteria=u2 > Threshold
  Wrap-up_Threshold : Constant  Value=wrap_up_threshold
  Wrap-up_Threshold1 : Constant  Value=basic_cycle_duration
  Out1 : Outport
  wires:
  Wrap-up_Threshold1/1 -> Minus/2
  Minus/1 -> Switch/1
  Switch/1 -> Out1/1
  GreaterThan/1 -> Switch/2
  Wrap-up_Threshold/1 -> GreaterThan/2
  In1/1 -> GreaterThan/1, Switch/3, Minus/1

== system HANcoder_E407_GTSync_v3_clean/HANcoder STM32 Target - E407-STM32 algorithm/Global Ticks Increment/CAN Management/CAN Recieve/CAN Receive System/Initialize message reception/Init_CAN_RX/CAN receive ==
  In1 : Inport
  Enabled Subsystem : Subsystem  TreatAsAtomicUnit=on
  S-Function : M-S-Function  FunctionName=sfcn_can_receive  Parameters=tsamp, canBus, outputNumber, dataType, byteOrder
  Out1 : Outport
  Out2 : Outport  Port=2
  Out3 : Outport  Port=3
  Out4 : Outport  Port=4
  Out5 : Outport  Port=5
  Out6 : Outport  Port=6
  Out7 : Outport  Port=7
  Out8 : Outport  Port=8
  Out9 : Outport  Port=9
  wires:
  In1/1 -> S-Function/1
  S-Function/1 -> Enabled Subsystem/Enable, Out1/1
  S-Function/2 -> Enabled Subsystem/1(In1)
  S-Function/3 -> Enabled Subsystem/2(In2)
  Enabled Subsystem/1(Out1) -> Out2/1
  Enabled Subsystem/2(Out2) -> Out3/1
  Enabled Subsystem/3(Out3) -> Out4/1
  Enabled Subsystem/4(Out4) -> Out5/1
  Enabled Subsystem/5(Out5) -> Out6/1
  Enabled Subsystem/6(Out6) -> Out7/1
  Enabled Subsystem/7(Out7) -> Out8/1
  Enabled Subsystem/8(Out8) -> Out9/1
  S-Function/6 -> Enabled Subsystem/5(In5)
  S-Function/7 -> Enabled Subsystem/6(In6)
  S-Function/8 -> Enabled Subsystem/7(In7)
  S-Function/5 -> Enabled Subsystem/4(In4)
  S-Function/4 -> Enabled Subsystem/3(In3)
  S-Function/9 -> Enabled Subsystem/8(In8)

== system HANcoder_E407_GTSync_v3_clean/HANcoder STM32 Target - E407-STM32 algorithm/Global Ticks Increment/CAN Management/CAN Recieve/CAN Receive System/Initialize message reception/Init_CAN_RX/Subsystem ==
  Initial Msg : Inport
  Enable : EnablePort
  Constant : Constant  Value=2
  Data Store Write : DataStoreWrite  DataStoreName=Local_Msg_Buffer  DataStoreElements=Local_Msg_Buffer.Buffer_1#Local_Msg_Buffer.Buffer_2#Local_Msg_Buffer.Buffer_3#Local_Msg_Buffer.Buffer_4#Local_Msg_Buffer.Buffer_5#Local_Msg_Buffer.Buffer_6#Local_Msg_Buffer.Buffer_7#Local_Msg_Buffer.Buffer_8
  Data Store Write1 : DataStoreWrite  DataStoreName=Init_CAN_RX_State
  Demux : Demux  Outputs=8
  wires:
  Constant/1 -> Data Store Write1/1
  Demux/1 -> Data Store Write/1
  Demux/2 -> Data Store Write/2
  Demux/3 -> Data Store Write/3
  Demux/4 -> Data Store Write/4
  Demux/5 -> Data Store Write/5
  Demux/6 -> Data Store Write/6
  Demux/7 -> Data Store Write/7
  Demux/8 -> Data Store Write/8
  Initial Msg/1 -> Demux/1

== system HANcoder_E407_GTSync_v3_clean/HANcoder STM32 Target - E407-STM32 algorithm/Global Ticks Increment/CAN Management/CAN Recieve/CAN Receive System/Initialize message reception/Init_CAN_RX/Subsystem1 ==
  Current Msg : Inport
  Enable : EnablePort
  Data Store Read2 : DataStoreRead  DataStoreName=Local_Msg_Buffer  DataStoreElements=Local_Msg_Buffer.Buffer_1#Local_Msg_Buffer.Buffer_2#Local_Msg_Buffer.Buffer_3#Local_Msg_Buffer.Buffer_4#Local_Msg_Buffer.Buffer_5#Local_Msg_Buffer.Buffer_6#Local_Msg_Buffer.Buffer_7#Local_Msg_Buffer.Buffer_8
  Demux : Demux  Outputs=8
  Equal{1..8} (8 alike) : RelationalOperator  Operator=~=  OutDataTypeStr=boolean  RndMeth=Simplest
  OR : Logic  Operator=OR  Inputs=8  IconShape=distinctive  AllPortsSameDT=off  OutDataTypeStr=boolean
  New and Different Msg : Outport
  wires:
  Current Msg/1 -> Demux/1
  Data Store Read2/1 -> Equal1/1
  Equal2/1 -> OR/2
  Equal3/1 -> OR/3
  Equal4/1 -> OR/4
  Equal5/1 -> OR/5
  Equal6/1 -> OR/6
  Equal7/1 -> OR/7
  Equal8/1 -> OR/8
  Equal1/1 -> OR/1
  OR/1 -> New and Different Msg/1
  Demux/1 -> Equal1/2
  Demux/3 -> Equal3/2
  Demux/4 -> Equal4/2
  Demux/5 -> Equal5/2
  Demux/6 -> Equal6/2
  Demux/7 -> Equal7/2
  Demux/8 -> Equal8/2
  Demux/2 -> Equal2/2
  Data Store Read2/2 -> Equal2/1
  Data Store Read2/3 -> Equal3/1
  Data Store Read2/4 -> Equal4/1
  Data Store Read2/5 -> Equal5/1
  Data Store Read2/6 -> Equal6/1
  Data Store Read2/7 -> Equal7/1
  Data Store Read2/8 -> Equal8/1

== system HANcoder_E407_GTSync_v3_clean/HANcoder STM32 Target - E407-STM32 algorithm/Global Ticks Increment/CAN Management/CAN Recieve/CAN Receive System/Subsystem/CAN receive/Enabled Subsystem ==
  In1 : Inport
  In2 : Inport  Port=2
  In3 : Inport  Port=3
  In4 : Inport  Port=4
  In5 : Inport  Port=5
  In6 : Inport  Port=6
  In7 : Inport  Port=7
  In8 : Inport  Port=8
  Enable : EnablePort
  Out1 : Outport
  Out2 : Outport  Port=2
  Out3 : Outport  Port=3
  Out4 : Outport  Port=4
  Out5 : Outport  Port=5
  Out6 : Outport  Port=6
  Out7 : Outport  Port=7
  Out8 : Outport  Port=8
  wires:
  In8/1 -> Out8/1
  In7/1 -> Out7/1
  In6/1 -> Out6/1
  In5/1 -> Out5/1
  In4/1 -> Out4/1
  In3/1 -> Out3/1
  In2/1 -> Out2/1
  In1/1 -> Out1/1

== system HANcoder_E407_GTSync_v3_clean/HANcoder STM32 Target - E407-STM32 algorithm/Global Ticks Increment/CAN Management/CAN Recieve/CAN Receive System/Subsystem1/CAN receive/Enabled Subsystem ==
  In1 : Inport
  In2 : Inport  Port=2
  In3 : Inport  Port=3
  In4 : Inport  Port=4
  In5 : Inport  Port=5
  In6 : Inport  Port=6
  In7 : Inport  Port=7
  In8 : Inport  Port=8
  Enable : EnablePort
  Out1 : Outport
  Out2 : Outport  Port=2
  Out3 : Outport  Port=3
  Out4 : Outport  Port=4
  Out5 : Outport  Port=5
  Out6 : Outport  Port=6
  Out7 : Outport  Port=7
  Out8 : Outport  Port=8
  wires:
  In1/1 -> Out1/1
  In2/1 -> Out2/1
  In3/1 -> Out3/1
  In4/1 -> Out4/1
  In5/1 -> Out5/1
  In6/1 -> Out6/1
  In7/1 -> Out7/1
  In8/1 -> Out8/1

== system HANcoder_E407_GTSync_v3_clean/HANcoder STM32 Target - E407-STM32 algorithm/Global Ticks Increment/CAN Management/CAN Recieve/CAN Receive System/Subsystem2/CAN receive/Enabled Subsystem ==
  In1 : Inport
  In2 : Inport  Port=2
  In3 : Inport  Port=3
  In4 : Inport  Port=4
  In5 : Inport  Port=5
  In6 : Inport  Port=6
  In7 : Inport  Port=7
  In8 : Inport  Port=8
  Enable : EnablePort
  Out1 : Outport
  Out2 : Outport  Port=2
  Out3 : Outport  Port=3
  Out4 : Outport  Port=4
  Out5 : Outport  Port=5
  Out6 : Outport  Port=6
  Out7 : Outport  Port=7
  Out8 : Outport  Port=8
  wires:
  In8/1 -> Out8/1
  In7/1 -> Out7/1
  In6/1 -> Out6/1
  In5/1 -> Out5/1
  In4/1 -> Out4/1
  In3/1 -> Out3/1
  In2/1 -> Out2/1
  In1/1 -> Out1/1
